simulink model "BEVModel"  (R2023a)
settings: Solver=VariableStepAuto  StartTime=0.0  StopTime=10.0  RelTol=1e-3
undefined symbols (not defined in the file or in its folder): Ion, Lithium
libraries: autolibshared x2, spsBatteryLib x1
settings Model: Creator=koush  LastModifiedBy=koush

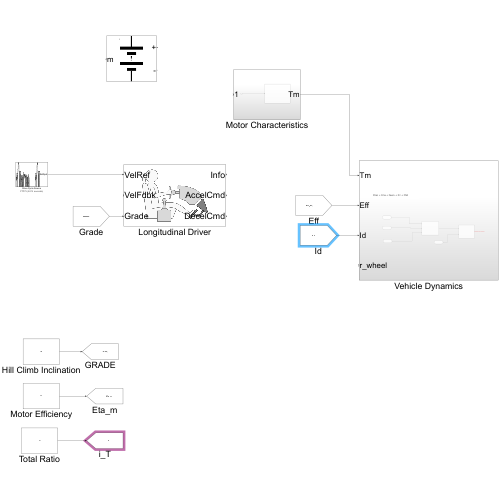
[thumbnail: Simulink's stored preview of the top-level diagram]
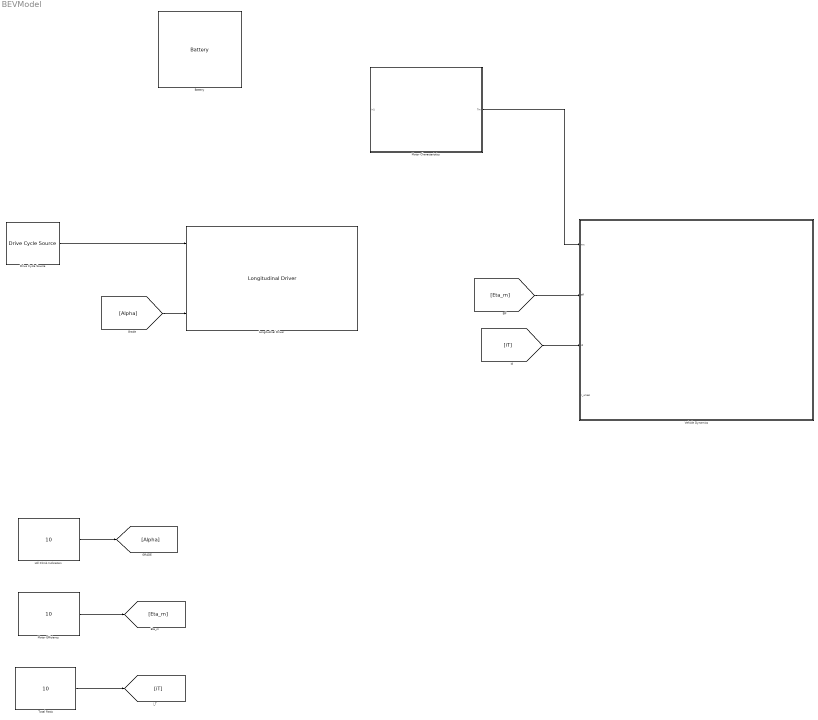
== system BEVModel ==
  Battery : spsBatteryLib/Battery  BatType=Lithium-Ion  ShowTempParam=off  ThermalPreset=no  ShowAgeParam=off  NomV=7.2  NomQ=5.4  SOC=100  Batt_Tr=30  PresetModel=on  MaxQ=5.4  MinV=5.4  FullV=8.3807  Dis_rate=2.3478  R=0.013333  Normal_OP=4.8835  expZone="[7.7788      0.2653]"  current=[6.5 13 32.5]  Units=Time  Tci=20  NomT=20  T2=-30  MaxQ2=4.8  FullV2=7.1  Normal_OP2=5.655  expZone2="[6.58           1]"  Rca=0.6  ti=2000  Dp=0  Neq0=0  Tsim=1e6  Ta1=25  Qeol=5.4*0.9  Reol=0.013333*1.2  Char_age=[2.3478, 3]  Dis_age=[2.3478, 10]  N1=1500  N2=10500  N3=1000  N4=1400  Ta2=45  N5=950
  Drive Cycle Source : autolibshared/Drive Cycle Source  cycleVar=FTP75  fileVar=cycleFTP75.mat  tfinal="2474  seconds"  cycleRepeat=off  outAccPort=off  outGearPort=off  gearList=No gear data  t_wot1=5  xdot_woto=0  xdot_wot1=30  t_wot2=20  xdot_wot2=0  t_wotend=30  srcUnit=m/s  outUnit=m/s  srcAccUnit=m/s/s  outAccUnit=m/s^2  dt=0  aMode=1  faultOption=off  velBnd=2  velBndUnit=mph  inUnit=m/s  timeBnd=1  failOption=off  stopSim=off  maxFaultCnt=10  maxFaultTime=2  maxTotFaultTime=15  traceOption=off  dtTrace=1  traceWindow=10  lastDCname=FTP75  lastOutUnit=mph  lastDT=0  lastTB=1  lastSB=2  forceCalcBound=off
  Hill Climb Inclination : Constant  Value=10
  Longitudinal Driver : autolibshared/Longitudinal Driver  extAccelOvr=off  extDecelOvr=off  extAccelHld=off  extDecelHld=off  extAccelZero=off  extDecelZero=off  cntrlType=PI  shftType=None  velUnits=m/s  gearOut=off  Kp=15  Ki=1  Kff=.05  Kg=.01  VehVelVec=[0 100]  KffVec=[.1 .1]  KpVec=[10 10]  KiVec=[5 5]  KgVec=[0 0]  m=1500  Kpt=3000  tau=.1  L=2  aR=200  bR=2.5  cR=.5  g=9.81  vnom=100  Kaw=.1  tauerr=.03  tauPt=2  GearInit=0  tShift=.1  pdlVec=[0.1 0.4 0.5 0.9]  upShftTbl=[-1 12.9375 26.4375 39.9375 51.18749999999999 62.4375 72.84375 83.25;-1 16.3125 29.8125 43.3125 54.5624 65.8125 76.78125 87.75;-1 19.6875 33.1875 46.68749999999999 57.9375 69.1875 80.71875 92.25;-1 33 52.5 77.25 100.5 138.75 161.875 185]  dwnShftTbl=[1 9.5625 23.0625 36.5625 47.8125 59.0625 68.90625 78.75;1 12.9375 26.4375 39.9375 51.18749999999999 62.4375 72.84375 83.25;1 16.3125 29.8125 43.3125 54.562499 65.8125 76.78125 87.75;1 19.6875 33.1875 46.68749999999999 57.9375 69.1875 80.71875 92.25]  tClutch=.5  tRev=.5  tPark=120  aMode=1  UpGearVec="[0  1  2  3  4  5  6  7]"  DownGearVec="[1  2  3  4  5  6  7  8]"
  Motor Characteristics : Subsystem
  Motor Efficiency : Constant  Value=10
  Total Ratio : Constant  Value=10
  Vehicle Dynamics : Subsystem
  wires:
  [Alpha] -> Longitudinal Driver/3
  Hill Climb Inclination/1 -> [Alpha]
  Drive Cycle Source/1 -> Longitudinal Driver/1
  Motor Efficiency/1 -> [Eta_m]
  Total Ratio/1 -> [iT]
  [Eta_m] -> Vehicle Dynamics/2(Eff)
  [iT] -> Vehicle Dynamics/3(Id)
  Motor Characteristics/1(Tm) -> Vehicle Dynamics/1(Tm)

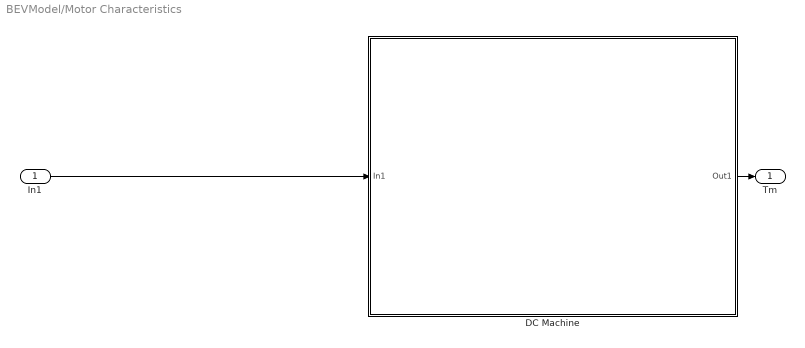
== system BEVModel/Motor Characteristics ==
  In1 : Inport
  DC Machine : Subsystem
  Tm : Outport
  wires:
  In1/1 -> DC Machine/1(In1)
  DC Machine/1(Out1) -> Tm/1

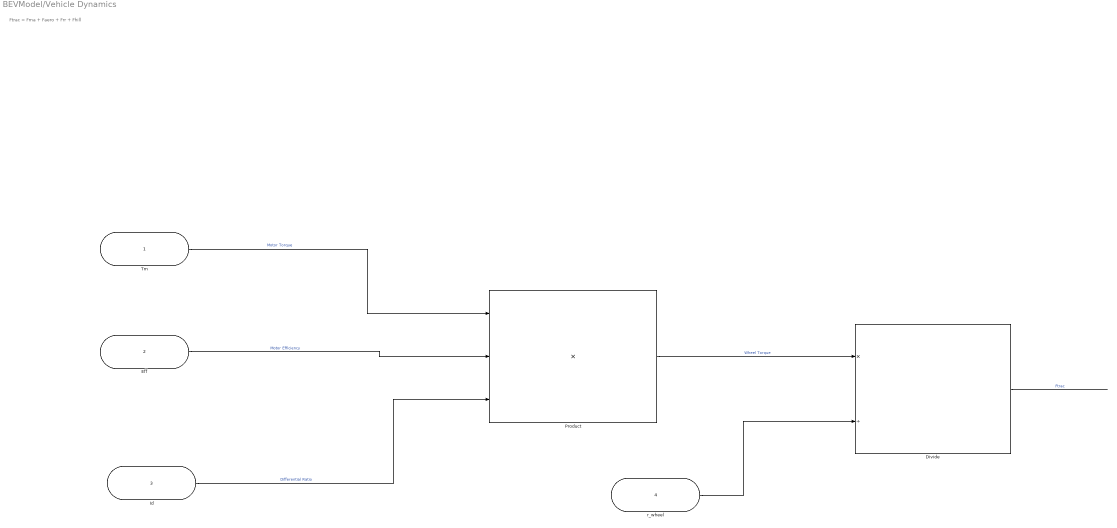
== system BEVModel/Vehicle Dynamics ==
  note: Ftrac = Fma + Faero + Frr + Fhill
  Tm : Inport
  Eff : Inport  Port=2
  Id : Inport  Port=3
  r_wheel : Inport  Port=4
  Divide : Product  Inputs=*/
  Product : Product  Inputs=3
  wires:
  Tm/1 -> Product/1  "Motor Torque"
  Eff/1 -> Product/2  "Motor Efficiency"
  Id/1 -> Product/3  "Differential Ratio"
  Product/1 -> Divide/1  "Wheel Torque"
  r_wheel/1 -> Divide/2
  Divide/1 -> ?  "Ftrac"

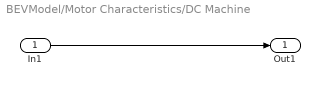
== system BEVModel/Motor Characteristics/DC Machine ==
  In1 : Inport
  Out1 : Outport
  wires:
  In1/1 -> Out1/1
